simulink model "system_identification"  (R2018a)
settings: Solver=VariableStepAuto  StartTime=0.0  StopTime=10.0  RelTol=1e-3
settings Model: Creator=thanhdo  LastModifiedBy=thanhdo

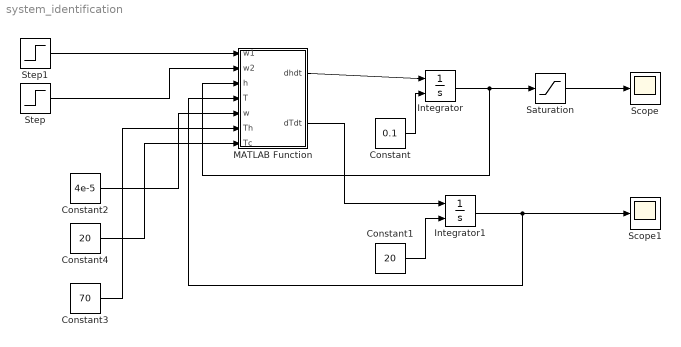
== system system_identification ==
  Constant : Constant  Value=0.1
  Constant1 : Constant  Value=20
  Constant2 : Constant  Value=4e-5
  Constant3 : Constant  Value=70
  Constant4 : Constant  Value=20
  Integrator : Integrator  InitialConditionSource=external
  Integrator1 : Integrator  InitialConditionSource=external
  MATLAB Function : MATLAB Function  TreatAsAtomicUnit=on
  Saturation : Saturate
  Scope : Scope
  Scope1 : Scope
  Step : Step  Time=0  Before=2e-5  SampleTime=0
  Step1 : Step  Time=0  Before=2e-5  SampleTime=0
  wires:
  Constant/1 -> Integrator/2
  Constant1/1 -> Integrator1/2
  Integrator1/1 -> MATLAB Function/4(T), Scope1/1
  Integrator/1 -> MATLAB Function/3(h), Saturation/1
  Step/1 -> MATLAB Function/2(w2)
  Step1/1 -> MATLAB Function/1(w1)
  MATLAB Function/1(dhdt) -> Integrator/1
  MATLAB Function/2(dTdt) -> Integrator1/1
  Constant2/1 -> MATLAB Function/5(w)
  Constant4/1 -> MATLAB Function/7(Tc)
  Constant3/1 -> MATLAB Function/6(Th)
  Saturation/1 -> Scope/1

== matlab function system_identification/MATLAB Function ==
  data: w1 input; dhdt output; w2 input; h input; T input; dTdt output; w input; Th input; Tc input
function [dhdt, dTdt] = fcn(w1, w2, h, T, w, Th, Tc)
A = 3.24e-2; %area of tank
dhdt = (w1 + w2 - w)/A;
dTdt = (w1*(Tc - T) - w2*(T - Th))/(A*h);
